simulink model "mdl01_IdealCtrl"  (R2022a)
settings: Solver=FixedStepAuto  StartTime=0.0  StopTime=T1  FixedStep=Ts  RelTol=1e-3
values from neighbouring files (symbols this model uses):
  a = 5    [Sim01_IdealCtrl.m]
  G1 = 1+K1*K2    [Sim01_IdealCtrl.m]
  G2 = K1+K2    [Sim01_IdealCtrl.m]
  Ts = 0.01    [Sim01_IdealCtrl.m]
  umax = 0.1    [Sim01_IdealCtrl.m]
  v0 = 0    [Sim01_IdealCtrl.m]
  x0 = -1    [Sim01_IdealCtrl.m]
settings Model: Creator=xiaocy  LastModifiedBy=xiaocy
settings DataIOCC: SaveOutput=off  SignalLogging=off  DSMLogging=off  SaveTime=off  ReturnWorkspaceOutputs=off

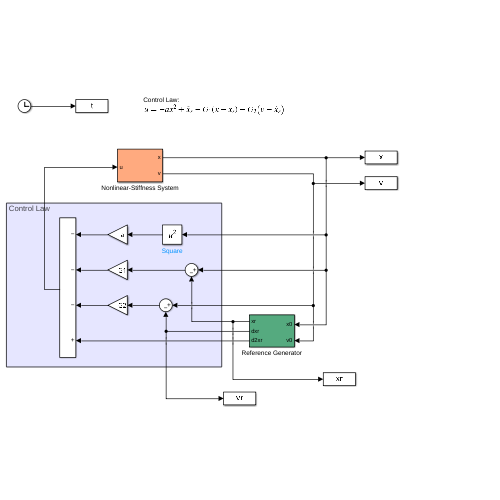
[thumbnail: Simulink's stored preview of the top-level diagram]
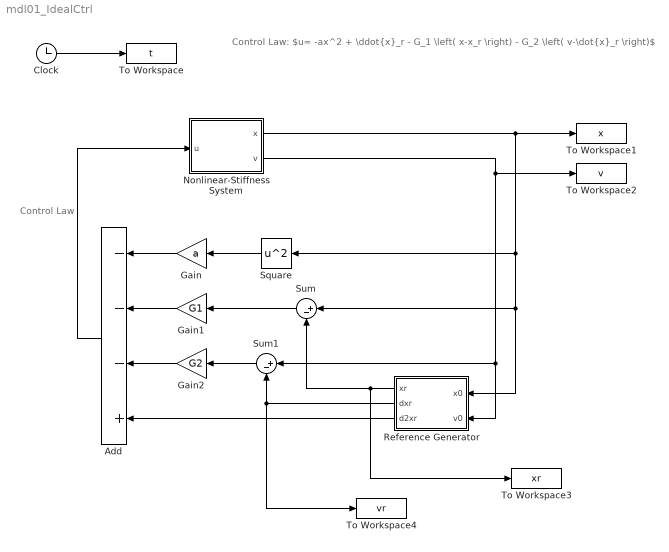
== system mdl01_IdealCtrl ==
  note: Control Law
  note: Control Law:
      | $u= -ax^2 + \ddot{x}_r - G_1 \left( x-x_r \right) - G_2 \left( v-\dot{x}_r \right)$
  Add : Sum  Inputs=---+
  Clock : Clock
  Gain : Gain  Gain=a
  Gain1 : Gain  Gain=G1
  Gain2 : Gain  Gain=G2
  Nonlinear-Stiffness System : Subsystem
  Reference Generator : Subsystem
  Square : Math  Operator=square
  Sum : Sum  Inputs=|+-
  Sum1 : Sum  Inputs=|+-
  To Workspace : ToWorkspace  VariableName=t  SampleTime=Ts
  To Workspace1 : ToWorkspace  VariableName=x  SampleTime=Ts
  To Workspace2 : ToWorkspace  VariableName=v  SampleTime=Ts
  To Workspace3 : ToWorkspace  VariableName=xr  SampleTime=Ts
  To Workspace4 : ToWorkspace  VariableName=vr  SampleTime=Ts
  wires:
  Clock/1 -> To Workspace/1
  Nonlinear-Stiffness System/1(x) -> Sum/1, Reference Generator/1(x0), Square/1, To Workspace1/1
  Nonlinear-Stiffness System/2(v) -> To Workspace2/1, Sum1/1, Reference Generator/2(v0)
  Reference Generator/1(xr) -> To Workspace3/1, Sum/2
  Sum/1 -> Gain1/1
  Sum1/1 -> Gain2/1
  Reference Generator/2(dxr) -> To Workspace4/1, Sum1/2
  Square/1 -> Gain/1
  Gain/1 -> Add/1
  Gain1/1 -> Add/2
  Gain2/1 -> Add/3
  Reference Generator/3(d2xr) -> Add/4
  Add/1 -> Nonlinear-Stiffness System/1(u)

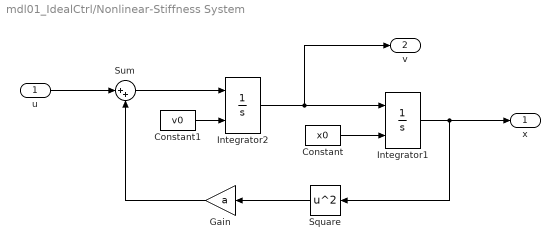
== system mdl01_IdealCtrl/Nonlinear-Stiffness System ==
  u : Inport
  Constant : Constant  Value=x0
  Constant1 : Constant  Value=v0
  Gain : Gain  Gain=a
  Integrator1 : Integrator  InitialConditionSource=external
  Integrator2 : Integrator  InitialConditionSource=external
  Square : Math  Operator=square
  Sum : Sum  Inputs=|++
  x : Outport
  v : Outport  Port=2
  wires:
  Gain/1 -> Sum/2
  Square/1 -> Gain/1
  Sum/1 -> Integrator2/1
  Integrator2/1 -> v/1, Integrator1/1
  u/1 -> Sum/1
  Integrator1/1 -> Square/1, x/1
  Constant/1 -> Integrator1/2
  Constant1/1 -> Integrator2/2

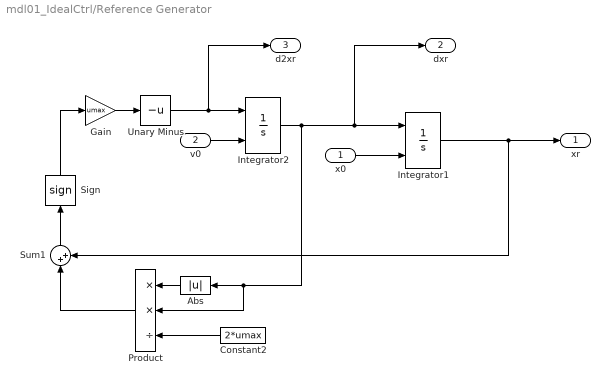
== system mdl01_IdealCtrl/Reference Generator ==
  x0 : Inport
  v0 : Inport  Port=2
  Abs : Abs  SaturateOnIntegerOverflow=off
  Constant2 : Constant  Value=2*umax
  Gain : Gain  Gain=umax
  Integrator1 : Integrator  InitialConditionSource=external
  Integrator2 : Integrator  InitialConditionSource=external
  Product : Product  Inputs=**/
  Sign : Signum
  Sum1 : Sum  Inputs=|++
  Unary Minus : UnaryMinus
  xr : Outport
  dxr : Outport  Port=2
  d2xr : Outport  Port=3
  wires:
  v0/1 -> Integrator2/2
  x0/1 -> Integrator1/2
  Integrator1/1 -> Sum1/2, xr/1
  Sum1/1 -> Sign/1
  Abs/1 -> Product/1
  Integrator2/1 -> Integrator1/1, dxr/1, Product/2, Abs/1
  Constant2/1 -> Product/3
  Product/1 -> Sum1/1
  Gain/1 -> Unary Minus/1
  Sign/1 -> Gain/1
  Unary Minus/1 -> d2xr/1, Integrator2/1
